simulink model "spike_generator"  (R2020b)
settings: Solver=FixedStepDiscrete  StartTime=0.0  StopTime=stopTime  RelTol=1e-3
values from neighbouring files (symbols this model uses):
  nSites = 4    [modelparameters.m]
  t_rd_init = t_rd_rest + 0.02e-3*spont - t_rd_jump    (= 0.0156)    [modelparameters.m]
  t_rd_jump = 0.4e-3    (= 0.0004)    [modelparameters.m]
  t_rd_rest = 14.0e-3    (= 0.014)    [modelparameters.m]
  tabs = 10e-3    (= 0.01)    [modelparameters.m]
  tau = 60e-3    (= 0.06)    [modelparameters.m]
  tdres = 1/Fs    (= 2.08333333333e-05)    [modelparameters.m]
  trel = 10e-3    (= 0.01)    [modelparameters.m]
undefined symbols (not defined in the file or in its folder): mp
libraries: hdlsllib x1
settings Model: Creator=Ross  LastModifiedBy=tyler
settings SolverCC: AutoInsertRateTranBlk=on
settings DataIOCC: SaveOutput=off  SaveTime=off  ReturnWorkspaceOutputs=off
settings OptimizationCC: BlockReduction=off  ConditionallyExecuteInputs=off  DefaultParameterBehavior=Inlined
settings DebuggingCC: ReadBeforeWriteMsg=DisableAll  WriteAfterWriteMsg=DisableAll  WriteAfterReadMsg=DisableAll  AlgebraicLoopMsg=error  MultiTaskDSMMsg=none  SingleTaskRateTransMsg=error  PregeneratedLibrarySubsystemCodeDiagnostic=none  ArithmeticOperatorsInVariantConditions=warning
settings HardwareCC: ProdBitPerPointer=32  ProdBitPerSizeT=32  ProdBitPerPtrDiffT=32  ProdLargestAtomicFloat=None  ProdIntDivRoundTo=Undefined  ProdEndianess=Unspecified  ProdWordSize=32  ProdHWDeviceType=ASIC/FPGA->ASIC/FPGA  TargetBitPerPointer=64  TargetBitPerSizeT=64  TargetBitPerPtrDiffT=64  TargetLongLongMode=on  TargetIntDivRoundTo=Zero  TargetEndianess=LittleEndian  TargetWordSize=64  TargetHWDeviceType=Custom Processor->MATLAB Host Computer  ProdEqTarget=off
settings ModelReferenceCC: UpdateModelReferenceTargets=IfOutOfDate  ModelReferenceNumInstancesAllowed=Single
settings SFSimCC: SFSimEcho=off  SimUseLocalCustomCode=off  CustomCodeUndefinedFunction=UseInterfaceOnly
settings RTWCC: RTWUseLocalCustomCode=off

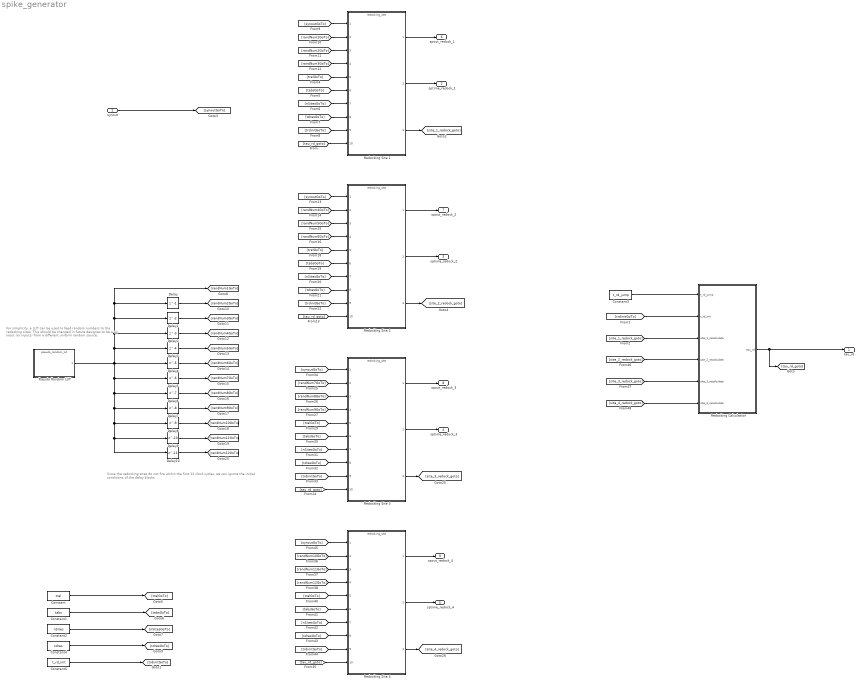
== system spike_generator ==
  note: For simplicity, a LUT can be used to feed random numbers to the redocking sites. This should be changed in future designes to be a an input (or inputs) from a different uniform random source.
  note: Since the redocking sites do not fire within the first 12 clock cycles, we can ignore the initial conditions of the delay blocks
  synout : Inport
  Constant : Constant  Value=trel  OutDataTypeStr=single  SampleTime=mp.Ts_sim
  Constant1 : Constant  Value=tabs  OutDataTypeStr=single  SampleTime=mp.Ts_sim
  Constant2 : Constant  Value=nSites  OutDataTypeStr=single  SampleTime=mp.Ts_sim
  Constant3 : Constant  Value=t_rd_jump  OutDataTypeStr=single  SampleTime=mp.Ts_sim
  Constant4 : Constant  Value=tdres  OutDataTypeStr=single  SampleTime=mp.Ts_sim
  Constant5 : Constant  Value=t_rd_init  OutDataTypeStr=single  SampleTime=mp.Ts_sim
  Delay : Delay  DelayLength=1
  Delay1 : Delay
  Delay10 : Delay  DelayLength=11
  Delay2 : Delay  DelayLength=3
  Delay3 : Delay  DelayLength=4
  Delay4 : Delay  DelayLength=5
  Delay5 : Delay  DelayLength=6
  Delay6 : Delay  DelayLength=7
  Delay7 : Delay  DelayLength=8
  Delay8 : Delay  DelayLength=9
  Delay9 : Delay  DelayLength=10
  Pseudo Random LUT : ModelReference  ModelNameDialog=pseudo_random_lut  SimulationMode=Normal  ModelReferenceVersion=1.295
  Redocking Calculation : Subsystem
  Redocking Site {1..4} (4 alike) : ModelReference  ModelNameDialog=redocking_site  SimulationMode=Normal  ModelReferenceVersion=1.299
  tau_rd : Outport
  sptime_redock_1 : Outport  Port=2
  sptime_redock_2 : Outport  Port=3
  sptime_redock_3 : Outport  Port=4
  sptime_redock_4 : Outport  Port=5
  spout_redock_1 : Outport  Port=6
  spout_redock_2 : Outport  Port=7
  spout_redock_3 : Outport  Port=8
  spout_redock_4 : Outport  Port=9
  wires:
  [tau_rd_goto] -> Redocking Site 1/10
  Redocking Site 1/3 -> [site_1_redock_goto]
  Constant3/1 -> Redocking Calculation/1(t_rd_jump)
  [trdinitGoTo] -> Redocking Calculation/2(t_rd_init)
  Redocking Site 1/1 -> spout_redock_1/1
  Redocking Site 1/2 -> sptime_redock_1/1
  Constant5/1 -> [trdinitGoTo]
  [site_1_redock_goto] -> Redocking Calculation/3(site_1_recalculate)
  Redocking Calculation/1(tau_rd) -> tau_rd/1, [tau_rd_goto]
  synout/1 -> [synoutGoTo]
  Constant/1 -> [trelGoTo]
  Constant1/1 -> [tabsGoTo]
  Constant2/1 -> [nSitesGoTo]
  Constant4/1 -> [tdresGoTo]
  [trelGoTo] -> Redocking Site 1/5
  [tabsGoTo] -> Redocking Site 1/6
  [nSitesGoTo] -> Redocking Site 1/7
  [tdresGoTo] -> Redocking Site 1/8
  [trdinitGoTo] -> Redocking Site 1/9
  [synoutGoTo] -> Redocking Site 1/1
  [randNum1GoTo] -> Redocking Site 1/2
  [randNum2GoTo] -> Redocking Site 1/3
  [randNum3GoTo] -> Redocking Site 1/4
  [randNum4GoTo] -> Redocking Site 2/2
  [tdresGoTo] -> Redocking Site 2/8
  [nSitesGoTo] -> Redocking Site 2/7
  [trdinitGoTo] -> Redocking Site 2/9
  [tabsGoTo] -> Redocking Site 2/6
  Redocking Site 2/2 -> sptime_redock_2/1
  Redocking Site 2/3 -> [site_2_redock_goto]
  [tau_rd_goto] -> Redocking Site 2/10
  Redocking Site 2/1 -> spout_redock_2/1
  [trelGoTo] -> Redocking Site 2/5
  [randNum5GoTo] -> Redocking Site 2/3
  [randNum6GoTo] -> Redocking Site 2/4
  [synoutGoTo] -> Redocking Site 2/1
  Redocking Site 3/1 -> spout_redock_3/1
  [synoutGoTo] -> Redocking Site 3/1
  [randNum8GoTo] -> Redocking Site 3/3
  [randNum9GoTo] -> Redocking Site 3/4
  [trelGoTo] -> Redocking Site 3/5
  [tau_rd_goto] -> Redocking Site 3/10
  [tabsGoTo] -> Redocking Site 3/6
  [nSitesGoTo] -> Redocking Site 3/7
  [tdresGoTo] -> Redocking Site 3/8
  Redocking Site 3/3 -> [site_3_redock_goto]
  [trdinitGoTo] -> Redocking Site 3/9
  [randNum7GoTo] -> Redocking Site 3/2
  Redocking Site 3/2 -> sptime_redock_3/1
  Redocking Site 4/1 -> spout_redock_4/1
  [synoutGoTo] -> Redocking Site 4/1
  [randNum11GoTo] -> Redocking Site 4/3
  [randNum12GoTo] -> Redocking Site 4/4
  [trelGoTo] -> Redocking Site 4/5
  [tau_rd_goto] -> Redocking Site 4/10
  [tabsGoTo] -> Redocking Site 4/6
  [nSitesGoTo] -> Redocking Site 4/7
  [tdresGoTo] -> Redocking Site 4/8
  Redocking Site 4/3 -> [site_4_redock_goto]
  [trdinitGoTo] -> Redocking Site 4/9
  [randNum10GoTo] -> Redocking Site 4/2
  Redocking Site 4/2 -> sptime_redock_4/1
  [site_3_redock_goto] -> Redocking Calculation/5(site_3_recalculate)
  [site_2_redock_goto] -> Redocking Calculation/4(site_2_recalculate)
  [site_4_redock_goto] -> Redocking Calculation/6(site_4_recalculate)
  Pseudo Random LUT/1 -> Delay3/1, Delay2/1, Delay1/1, Delay/1, [randNum1GoTo], Delay5/1, Delay10/1, Delay9/1, Delay8/1, Delay7/1, Delay6/1, Delay4/1
  Delay1/1 -> [randNum3GoTo]
  Delay/1 -> [randNum2GoTo]
  Delay7/1 -> [randNum9GoTo]
  Delay8/1 -> [randNum10GoTo]
  Delay9/1 -> [randNum11GoTo]
  Delay10/1 -> [randNum12GoTo]
  Delay6/1 -> [randNum8GoTo]
  Delay5/1 -> [randNum7GoTo]
  Delay4/1 -> [randNum6GoTo]
  Delay3/1 -> [randNum5GoTo]
  Delay2/1 -> [randNum4GoTo]

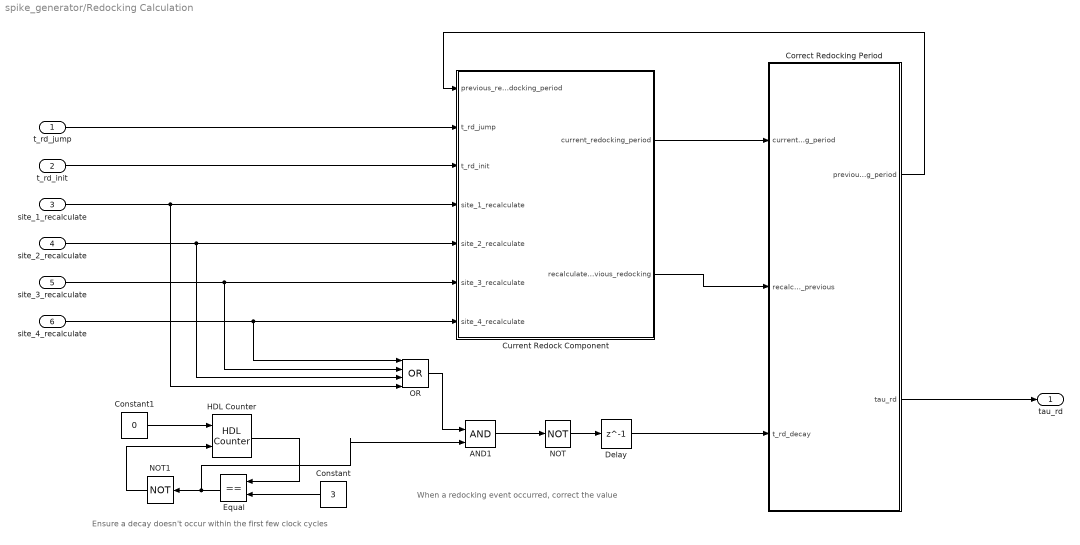
== system spike_generator/Redocking Calculation ==
  note: When a redocking event occurred, correct the value
  note: Ensure a decay doesn't occur within the first few clock cycles
  t_rd_jump : Inport
  t_rd_init : Inport  Port=2
  site_1_recalculate : Inport  Port=3
  site_2_recalculate : Inport  Port=4
  site_3_recalculate : Inport  Port=5
  site_4_recalculate : Inport  Port=6
  AND1 : Logic  IconShape=distinctive  AllPortsSameDT=off  OutDataTypeStr=boolean
  Constant : Constant  Value=3  OutDataTypeStr=int8  SampleTime=-1
  Constant1 : Constant  Value=0  OutDataTypeStr=boolean  SampleTime=-1
  Correct Redocking Period : Subsystem
  Current Redock Component : Subsystem
  Delay : Delay  DelayLength=1
  Equal : RelationalOperator  Operator===  OutDataTypeStr=boolean  RndMeth=Simplest
  HDL Counter : hdlsllib/Sources/HDL Counter  CountType=Count limited  CountInit=0  CountStep=1  CountMax=3  CountFromType=Initial value  CountFrom=0  CountResetPort=on  CountLoadPort=off  CountEnbPort=on  CountDirPort=off  CountDataType=Unsigned  CountWordLen=8  CountFracLen=0  CountSampTime=-1
  NOT : Logic  Operator=NOT  IconShape=distinctive  AllPortsSameDT=off  OutDataTypeStr=boolean
  NOT1 : Logic  Operator=NOT  IconShape=distinctive  AllPortsSameDT=off  OutDataTypeStr=boolean
  OR : Logic  Operator=OR  Inputs=4  IconShape=distinctive  AllPortsSameDT=off  OutDataTypeStr=boolean
  tau_rd : Outport  InitialOutput=0
  wires:
  t_rd_init/1 -> Current Redock Component/3(t_rd_init)
  t_rd_jump/1 -> Current Redock Component/2(t_rd_jump)
  Current Redock Component/1(current_redocking_period) -> Correct Redocking Period/1(current_redocking_period)
  site_1_recalculate/1 -> OR/4, Current Redock Component/4(site_1_recalculate)
  Current Redock Component/2(recalculate_previous_redocking) -> Correct Redocking Period/2(recalculate_previous)
  site_2_recalculate/1 -> OR/3, Current Redock Component/5(site_2_recalculate)
  site_3_recalculate/1 -> OR/2, Current Redock Component/6(site_3_recalculate)
  site_4_recalculate/1 -> OR/1, Current Redock Component/7(site_4_recalculate)
  Delay/1 -> Correct Redocking Period/3(t_rd_decay)
  NOT/1 -> Delay/1
  Constant1/1 -> HDL Counter/1
  OR/1 -> AND1/1
  HDL Counter/1 -> Equal/1
  AND1/1 -> NOT/1
  NOT1/1 -> HDL Counter/2
  Correct Redocking Period/1(previous_redocking_period) -> Current Redock Component/1(previous_redocking_period)
  Correct Redocking Period/2(tau_rd) -> tau_rd/1
  Equal/1 -> AND1/2, NOT1/1
  Constant/1 -> Equal/2

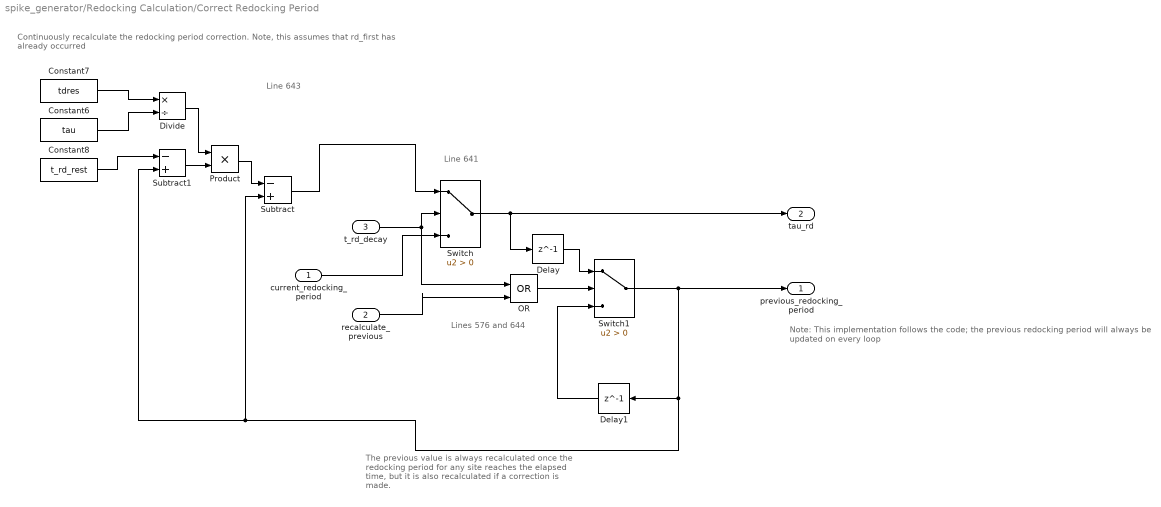
== system spike_generator/Redocking Calculation/Correct Redocking Period ==
  note: Note: This implementation follows the code; the previous redocking period will always be updated on every loop
  note: The previous value is always recalculated once the redocking period for any site reaches the elapsed time, but it is also recalculated if a correction is made.
  note: Lines 576 and 644
  note: Continuously recalculate the redocking period correction. Note, this assumes that rd_first has already occurred
  note: Line 643
  note: Line 641
  current_redocking_period : Inport
  recalculate_previous : Inport  Port=2
  t_rd_decay : Inport  Port=3
  Constant6 : Constant  Value=tau  OutDataTypeStr=single  SampleTime=-1
  Constant7 : Constant  Value=tdres  OutDataTypeStr=single  SampleTime=-1
  Constant8 : Constant  Value=t_rd_rest  OutDataTypeStr=single  SampleTime=-1
  Delay : Delay  DelayLength=1
  Delay1 : Delay  DelayLength=1
  Divide : Product  Inputs=*/
  OR : Logic  Operator=OR  IconShape=distinctive  AllPortsSameDT=off  OutDataTypeStr=boolean
  Product : Product
  Subtract : Sum  Inputs=-+
  Subtract1 : Sum  Inputs=-+
  Switch : Switch  Criteria=u2 > Threshold
  Switch1 : Switch  Criteria=u2 > Threshold
  previous_redocking_period : Outport
  tau_rd : Outport  Port=2
  wires:
  Product/1 -> Subtract/1
  Subtract1/1 -> Product/2
  Divide/1 -> Product/1
  Constant6/1 -> Divide/2
  Constant7/1 -> Divide/1
  Switch/1 -> tau_rd/1, Delay/1
  t_rd_decay/1 -> Switch/2, OR/1
  Delay1/1 -> Switch1/3
  Delay/1 -> Switch1/1
  OR/1 -> Switch1/2
  recalculate_previous/1 -> OR/2
  Switch1/1 -> Subtract1/2, Subtract/2, Delay1/1, previous_redocking_period/1
  Subtract/1 -> Switch/1
  current_redocking_period/1 -> Switch/3
  Constant8/1 -> Subtract1/1

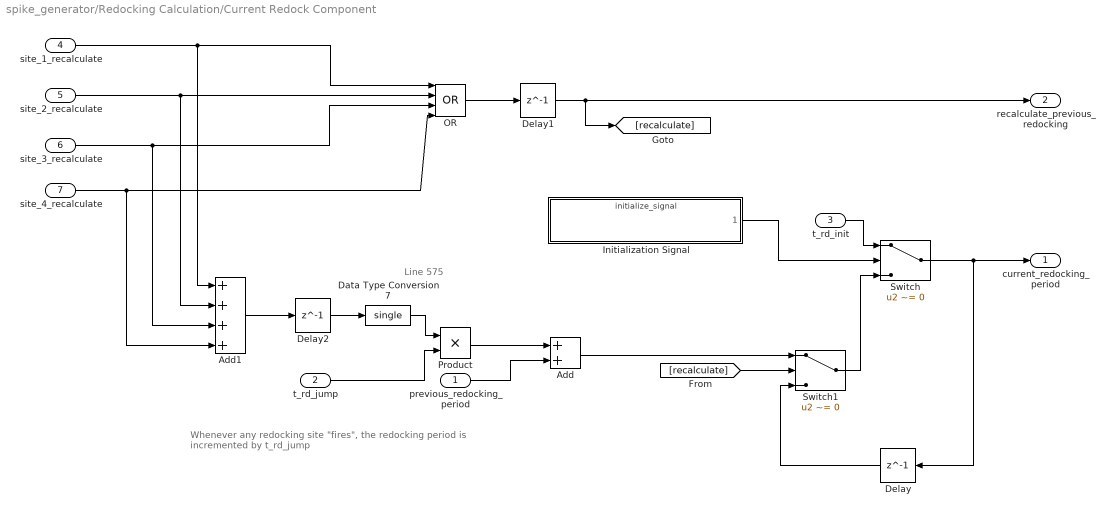
== system spike_generator/Redocking Calculation/Current Redock Component ==
  note: Whenever any redocking site "fires", the redocking period
      | is incremented by t_rd_jump
  note: Line 575
  previous_redocking_period : Inport
  t_rd_jump : Inport  Port=2
  t_rd_init : Inport  Port=3
  site_1_recalculate : Inport  Port=4
  site_2_recalculate : Inport  Port=5
  site_3_recalculate : Inport  Port=6
  site_4_recalculate : Inport  Port=7
  Add : Sum
  Add1 : Sum  Inputs=++++
  Data Type Conversion7 : DataTypeConversion  OutDataTypeStr=single  RndMeth=Nearest
  Delay : Delay  DelayLength=1
  Delay1 : Delay  DelayLength=1
  Delay2 : Delay  DelayLength=1
  Initialization Signal : ModelReference  ModelNameDialog=initialize_signal  SimulationMode=Normal  ModelReferenceVersion=1.282
  OR : Logic  Operator=OR  Inputs=4  IconShape=distinctive  AllPortsSameDT=off  OutDataTypeStr=boolean
  Product : Product
  Switch : Switch  Criteria=u2 ~= 0  OutDataTypeStr=single
  Switch1 : Switch  Criteria=u2 ~= 0  OutDataTypeStr=single
  current_redocking_period : Outport
  recalculate_previous_redocking : Outport  Port=2
  wires:
  Switch/1 -> current_redocking_period/1, Delay/1
  Add/1 -> Switch1/1
  Switch1/1 -> Switch/3
  t_rd_init/1 -> Switch/1
  Initialization Signal/1 -> Switch/2
  site_1_recalculate/1 -> OR/1, Add1/1
  site_2_recalculate/1 -> OR/2, Add1/2
  site_3_recalculate/1 -> OR/3, Add1/3
  site_4_recalculate/1 -> OR/4, Add1/4
  previous_redocking_period/1 -> Add/2
  Product/1 -> Add/1
  t_rd_jump/1 -> Product/2
  Add1/1 -> Delay2/1
  OR/1 -> Delay1/1
  Delay1/1 -> recalculate_previous_redocking/1, [recalculate]
  Delay2/1 -> Data Type Conversion7/1
  Data Type Conversion7/1 -> Product/1
  Delay/1 -> Switch1/3
  [recalculate] -> Switch1/2
